simulink model "OOK_model3"  (Simulink 7.6)
settings: Solver=FixedStepDiscrete  SolverMode=SingleTasking  StartTime=0.0  StopTime=1  FixedStep=1/100000  RelTol=1e-3  AbsTol=1e-6
libraries: commchan3 x1, dsparch4 x1, simulink x1, commsink2 x1, commrandsrc2 x1
settings Model: Creator=hsalgado  LastModifiedBy=Sílvio  ExtModeAutoUpdateStatusClock=off
settings DataIOCC: LimitDataPoints=off
settings OptimizationCC: BlockReduction=off  BooleanDataType=off  InitFltsAndDblsToZero=on
settings DebuggingCC: SaveWithParameterizedLinksMsg=none  SignalResolutionControl=TryResolveAllWithWarning  SolverPrmCheckMsg=none  MultiTaskDSMMsg=warning  MultiTaskCondExecSysMsg=none  StrictBusMsg=None
settings HardwareCC: TargetUnknown=on
settings RTWCC: TemplateMakefile=grt_unix.tmf  IncludeERTFirstTime=on
settings GRTTargetCC: TargetFcnLib=ansi_tfl_tmw.mat  ModelReferenceCompliant=off  MatFileLogging=off

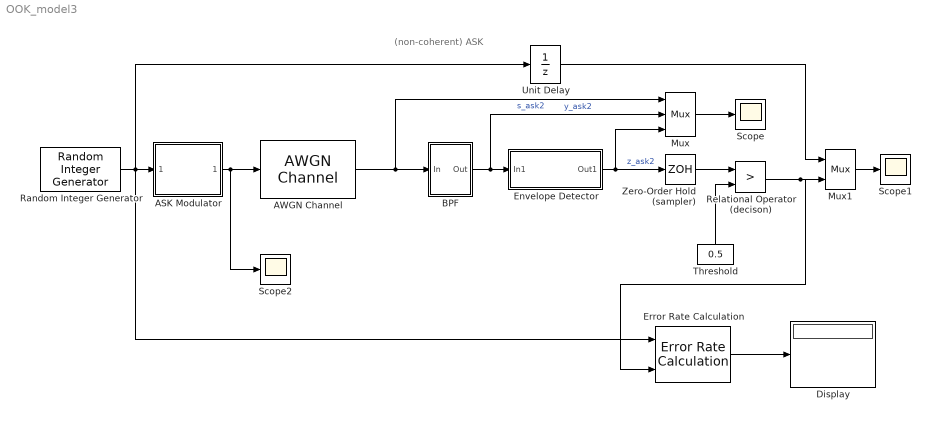
== system OOK_model3 ==
  note: (non-coherent) ASK
  ASK Modulator : Subsystem
  AWGN Channel : commchan3/AWGN Channel  SystemSampleTime=-1  InputProcessing=Inherited (this choice will be removed - see release notes)  seed=67  noiseMode=Variance from mask  EbNodB=10  EsNodB=10  SNRdB=10  bitsPerSym=1  Ps=1  Tsym=1  variance=1
  BPF : Subsystem
  Display : Display
  Envelope Detector : Subsystem  mask{g=1}
      mask prompts: g "Upper/Lower"
      mask Display: disp('Envelope\n detector')
  Error Rate Calculation : commsink2/Error Rate Calculation  N=1  st_delay=0  cp_mode=Entire frame  subframe=[]  PMode=Port  WsName=ErrorVec  RsMode2=off  stop=off  numErr=100  maxBits=1e6
  Mux : Mux  Inputs=3
  Mux1 : Mux  Inputs=2
  Random Integer Generator : commrandsrc2/Random Integer Generator  SystemSampleTime=-1  mul=2  seed=37  Ts=1/1000  frameBased=off  sampPerFrame=1  orient=off  outDataType=double
  Relational Operator (decison) : RelationalOperator  Operator=>  InputSameDT=on
  Scope : Scope
      settings: TickLabels=on  TimeRange=0.1  DataFormat=Array
  Scope1 : Scope
      settings: TickLabels=on  YMin=-2  YMax=2  DataFormat=Array
  Scope2 : Scope
      settings: TickLabels=on  YMin=-1  YMax=1  DataFormat=Array
  Threshold : Constant  Value=0.5
  Unit Delay : UnitDelay  SampleTime=1/1000
  Zero-Order Hold (sampler) : ZeroOrderHold  SampleTime=1/1000
  wires:
  Zero-Order Hold (sampler)/1 -> Relational Operator (decison)/1
  Envelope Detector/1(Out1) -> Mux/3, Zero-Order Hold (sampler)/1  "z_ask2"
  BPF/1(Out) -> Mux/2, Envelope Detector/1(In1)  "y_ask2"
  Unit Delay/1 -> Mux1/1
  Random Integer Generator/1 -> Unit Delay/1, ASK Modulator/1(Data in), Error Rate Calculation/1
  Mux1/1 -> Scope1/1
  Threshold/1 -> Relational Operator (decison)/2
  ASK Modulator/1(Carrier) -> AWGN Channel/1, Scope2/1
  Mux/1 -> Scope/1
  Relational Operator (decison)/1 -> Mux1/2, Error Rate Calculation/2
  AWGN Channel/1 -> Mux/1, BPF/1(In)  "s_ask2"
  Error Rate Calculation/1 -> Display/1

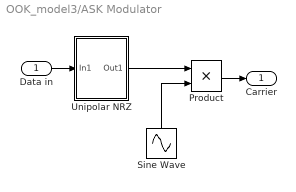
== system OOK_model3/ASK Modulator ==
  Data in : Inport
  Product : Product  SaturateOnIntegerOverflow=on  RndMeth=Zero  InputSameDT=on  OutDataTypeStr=Inherit: Same as first input
  Sine Wave : Sin  Frequency=2*pi*10000  SampleTime=0
  Unipolar NRZ : Subsystem
      mask Type: Unipolar NRZ
      mask Description:
      | This block encodes a signal into the unipolar NRZ line code
      | 
      | The output values are +1 for a nonzero input and zero otherwise.
      mask Display: disp('Unipolar\nNRZ')
  Carrier : Outport  InitialOutput=0
  wires:
  Product/1 -> Carrier/1
  Data in/1 -> Unipolar NRZ/1(In1)
  Unipolar NRZ/1(Out1) -> Product/1
  Sine Wave/1 -> Product/2

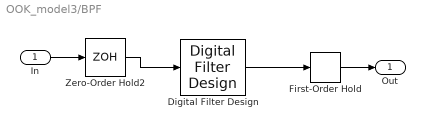
== system OOK_model3/BPF ==
  In : Inport
  Digital Filter Design : dsparch4/Digital Filter Design  SystemSampleTime=-1  mwdsp_browser_bugfix_var=off
  First-Order Hold : simulink/Discrete/First-Order Hold  SystemSampleTime=-1  Ts=1/100000
  Zero-Order Hold2 : ZeroOrderHold  SampleTime=1/100000
  Out : Outport  InitialOutput=0
  wires:
  Zero-Order Hold2/1 -> Digital Filter Design/1
  In/1 -> Zero-Order Hold2/1
  Digital Filter Design/1 -> First-Order Hold/1
  First-Order Hold/1 -> Out/1

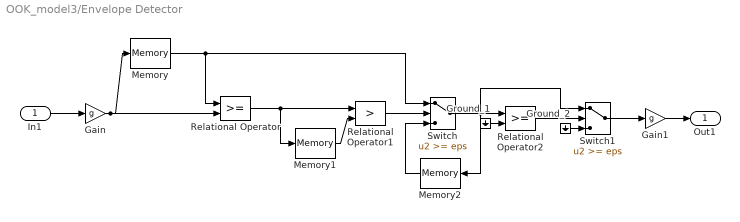
== system OOK_model3/Envelope Detector ==
  In1 : Inport
  Gain : Gain  Gain=g  SaturateOnIntegerOverflow=on  OutDataTypeStr=Inherit: Same as input  ParamDataTypeStr=Inherit: Same as input
  Gain1 : Gain  Gain=g  SaturateOnIntegerOverflow=on  OutDataTypeStr=Inherit: Same as input  ParamDataTypeStr=Inherit: Same as input
  Ground_1 : Ground
  Ground_2 : Ground
  Memory : Memory
  Memory1 : Memory
  Memory2 : Memory
  Relational Operator : RelationalOperator  InputSameDT=on
  Relational Operator1 : RelationalOperator  Operator=>  InputSameDT=on
  Relational Operator2 : RelationalOperator  InputSameDT=on
  Switch : Switch  Threshold=eps  SaturateOnIntegerOverflow=on  InputSameDT=on
  Switch1 : Switch  Threshold=eps  SaturateOnIntegerOverflow=on  InputSameDT=on
  Out1 : Outport
  wires:
  Gain1/1 -> Out1/1
  In1/1 -> Gain/1
  Ground_2/1 -> Switch1/3
  Ground_1/1 -> Relational Operator2/2
  Switch/1 -> Switch1/1, Memory2/1, Relational Operator2/1
  Relational Operator2/1 -> Switch1/2
  Switch1/1 -> Gain1/1
  Memory/1 -> Switch/1, Relational Operator/1
  Memory1/1 -> Relational Operator1/2
  Relational Operator/1 -> Relational Operator1/1, Memory1/1
  Relational Operator1/1 -> Switch/2
  Memory2/1 -> Switch/3
  Gain/1 -> Relational Operator/2, Memory/1

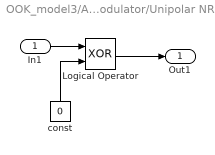
== system OOK_model3/ASK Modulator/Unipolar NRZ ==
  In1 : Inport
  Logical Operator : Logic  Operator=XOR
  const : Constant  Value=0
  Out1 : Outport  InitialOutput=0
  wires:
  Logical Operator/1 -> Out1/1
  In1/1 -> Logical Operator/1
  const/1 -> Logical Operator/2
